simulink library "SDTlibV1"  (R2025b)
settings: Solver=VariableStepAuto  StartTime=0.0  StopTime=10.0  RelTol=1e-3
PreLoadFcn:
  | addpath(genpath('SDTfct'));
values from neighbouring files (symbols this model uses):
  pass = ra2DCMi(blk.ra)    [view_SDTlib_model.m]
undefined symbols (not defined in the file or in its folder): CMG, DAP0, DPa0, FSM, Ignew, InvDyn, InvDynAug, Jr, KIN, kinematic_model, LS, Mdyn, mnew, mp, OGnew, PMA, ra_norm, RWS, sig4, uls, ureal, uss, uw, XI
libraries: RCTblocks x470, $bdroot x4
(part 4 of 10)

== system SDTlibV1/Space  subsystems/Four CMGs Pyramid ==
  Sigma_dot_ref : Inport
  m_at_P : Inport  Port=2
  CMG1 : Subsystem
  CMG2 : Subsystem
  CMG3 : Subsystem
  CMG4 : Subsystem
  Demux : Demux
  Mux : Mux
  P1/p : $bdroot/3//6 dof DCM/6x6 DCM  rot=[cos(CMG.alpha) -sin(CMG.alpha) 0;sin(CMG.alpha) cos(CMG.alpha) 0;0 0 1]*CMG.Pbeta  transp=off
  P1/p' : Subsystem  mask(18x18 Direction cosine matrix (DCM)){rot=[cos(CMG.alpha) -sin(CMG.alpha) 0;sin(CMG.alpha) cos(CMG.alpha) 0;0 0 1]*CMG.Pbeta, transp=on}
      mask prompts: rot "3x3 DCM"; transp "Matrix transposed"
      mask help:
      | For 6 d.o.f. body motion vector (3 translations and 3 rotations, acceleration velocities and positions), this block Implement the 18x18 rotation matrix (or its transposed) for a given 3x3 DCM.
      |
      | Considering 2 frames R1 and  R2, the DCM between R1 and R2 is defined as the 3x3 matrix where each column is the component vector of each R2 orthogonal unit vector expressed in R1. Thus
      |
      |    [v]_R1 = DCM  * [v]_R2.
      mask init:
      | if transp,
      |     rot=rot';
      | end
      mask Help: web('Doc6dcm.html','-browser','-browser')
      mask Display:
      | disp('18x18 DCM')
      | if transp
      |     port_label('input', 1, '[.]_R1')
      |     port_label('output', 1, '[.]_R2')
      | else
      |     port_label('input', 1, '[.]_R2')
      |     port_label('output', 1, '[.]_R1')
      | end
  P2/p : $bdroot/3//6 dof DCM/6x6 DCM  rot=[cos(CMG.alpha+pi/2) -sin(CMG.alpha+pi/2) 0;sin(CMG.alpha+pi/2) cos(CMG.alpha+pi/2) 0;0 0 1]*CMG.Pbeta  transp=off
  P2/p' : Subsystem  mask(18x18 Direction cosine matrix (DCM)){rot=[cos(CMG.alpha+pi/2) -sin(CMG.alpha+pi/2) 0;sin(CMG.alpha+pi/2) cos(CMG.alpha+pi/2) 0;0 0 1]*CMG.Pbeta, transp=on}
      mask prompts: rot "3x3 DCM"; transp "Matrix transposed"
      mask help:
      | For 6 d.o.f. body motion vector (3 translations and 3 rotations, acceleration velocities and positions), this block Implement the 18x18 rotation matrix (or its transposed) for a given 3x3 DCM.
      |
      | Considering 2 frames R1 and  R2, the DCM between R1 and R2 is defined as the 3x3 matrix where each column is the component vector of each R2 orthogonal unit vector expressed in R1. Thus
      |
      |    [v]_R1 = DCM  * [v]_R2.
      mask init:
      | if transp,
      |     rot=rot';
      | end
      mask Help: web('Doc6dcm.html','-browser','-browser')
      mask Display:
      | disp('18x18 DCM')
      | if transp
      |     port_label('input', 1, '[.]_R1')
      |     port_label('output', 1, '[.]_R2')
      | else
      |     port_label('input', 1, '[.]_R2')
      |     port_label('output', 1, '[.]_R1')
      | end
  P3/p : $bdroot/3//6 dof DCM/6x6 DCM  rot=[cos(CMG.alpha+pi) -sin(CMG.alpha+pi) 0;sin(CMG.alpha+pi) cos(CMG.alpha+pi) 0;0 0 1]*CMG.Pbeta  transp=off
  P3/p' : Subsystem  mask(18x18 Direction cosine matrix (DCM)){rot=[cos(CMG.alpha+pi) -sin(CMG.alpha+pi) 0;sin(CMG.alpha+pi) cos(CMG.alpha+pi) 0;0 0 1]*CMG.Pbeta, transp=on}
      mask prompts: rot "3x3 DCM"; transp "Matrix transposed"
      mask help:
      | For 6 d.o.f. body motion vector (3 translations and 3 rotations, acceleration velocities and positions), this block Implement the 18x18 rotation matrix (or its transposed) for a given 3x3 DCM.
      |
      | Considering 2 frames R1 and  R2, the DCM between R1 and R2 is defined as the 3x3 matrix where each column is the component vector of each R2 orthogonal unit vector expressed in R1. Thus
      |
      |    [v]_R1 = DCM  * [v]_R2.
      mask init:
      | if transp,
      |     rot=rot';
      | end
      mask Help: web('Doc6dcm.html','-browser','-browser')
      mask Display:
      | disp('18x18 DCM')
      | if transp
      |     port_label('input', 1, '[.]_R1')
      |     port_label('output', 1, '[.]_R2')
      | else
      |     port_label('input', 1, '[.]_R2')
      |     port_label('output', 1, '[.]_R1')
      | end
  P4/p : $bdroot/3//6 dof DCM/6x6 DCM  rot=[cos(CMG.alpha+3*pi/2) -sin(CMG.alpha+3*pi/2) 0;sin(CMG.alpha+3*pi/2) cos(CMG.alpha+3*pi/2) 0;0 0 1]*CMG.Pbeta  transp=off
  P4/p' : Subsystem  mask(18x18 Direction cosine matrix (DCM)){rot=[cos(CMG.alpha+3*pi/2) -sin(CMG.alpha+3*pi/2) 0;sin(CMG.alpha+3*pi/2) cos(CMG.alpha+3*pi/2) 0;0 0 1]*CMG.Pbeta, transp=on}
      mask prompts: rot "3x3 DCM"; transp "Matrix transposed"
      mask help:
      | For 6 d.o.f. body motion vector (3 translations and 3 rotations, acceleration velocities and positions), this block Implement the 18x18 rotation matrix (or its transposed) for a given 3x3 DCM.
      |
      | Considering 2 frames R1 and  R2, the DCM between R1 and R2 is defined as the 3x3 matrix where each column is the component vector of each R2 orthogonal unit vector expressed in R1. Thus
      |
      |    [v]_R1 = DCM  * [v]_R2.
      mask init:
      | if transp,
      |     rot=rot';
      | end
      mask Help: web('Doc6dcm.html','-browser','-browser')
      mask Display:
      | disp('18x18 DCM')
      | if transp
      |     port_label('input', 1, '[.]_R1')
      |     port_label('output', 1, '[.]_R2')
      | else
      |     port_label('input', 1, '[.]_R2')
      |     port_label('output', 1, '[.]_R1')
      | end
  massless connection body : Subsystem  mask(Massless multi_port [6+18(n-1)]x[6(n-1)+18]){n=5, numinv=5, OP1=[0;-CMG.r;0], OP2=[CMG.r;0;0], OP3=[0;CMG.r;0], OP4=[-CMG.r;0;0], OP5=[0;0;0], OP6=[0;0;0], OP7=[0;0;0]}
      mask prompts: n "Number of ports"; numinv "Port (point) Pj: j="; OP1 "OP1 (3x1 vector, m)"; OP2 "OP2 (3x1 vector, m)"; OP3 "OP3 (3x1 vector, m)"; OP4 "OP4 (3x1 vector, m)"; OP5 "OP5 (3x1 vector,m)"; OP6 "OP6 (3x1 vector,m)"; OP7 "OP7 (3x1 vector,m)"
      mask help:
      | Massless body to transport wrenches and acceleration twists:
      | [6+18(n-1)]x[6(n-1)+18] gain from:
      |  * the motion vector at one point Pj; i.e. the parent port,
      |  * the wrenches applied to this massless body at the n-1 points Pi (i=1,..n, except j); i.e. the child ports
      | to:
      |  * the wrench applied at point Pj by this massless body,
      |  * the motion vectors at the other n-1  points Pi (i=1,..n, except j).
      |
      | 0: the reference point
      | Pi (i=1:n): the n given connection points or ports (1<n<8).
      |
      | All parameters are expressed in the body frame.
      | Each parameter can be an uncertain parameter declared with "ureal"
      mask init:
      | MasslessConnectionBodyAug
      mask Help: %web('DocMassLessBody.html')
      mask TypeOptions n: 2 | 3 | 4 | 5 | 6 | 7
      mask TypeOptions numinv: 1 | 2 | 3 | 4 | 5 | 6 | 7
      mask DialogControl ParameterGroupVar Prompt: Main parameters
      mask DialogControl port1 Prompt: Port #1
      mask DialogControl port2 Prompt: #2
      mask DialogControl port3 Prompt: #3
      mask DialogControl port4 Prompt: #4
      mask DialogControl port5 Prompt: #5
      mask DialogControl port6 Prompt: #6
      mask DialogControl port7 Prompt: #7
      mask Display:
      | disp('Massless\n connection body\n [6+18(n-1)]x[6(n-1)+18]')
      | for ii=1:n+1
      |     if numinv==ii,
      |         port_label('output',ii,['W_body/.,P',num2str(ii)])
      |         port_label('input', ii,['m_P',num2str(ii)])
      |     else
      |         port_label('input', ii,['W_./body,P',num2str(ii)])
      |         port_label('output',ii,['m_P',num2str(ii)])
      |     end
      | end
  Sigma_dot : Outport
  W_CMGs/.,P : Outport  Port=2
  wires:
  Mux/1 -> Sigma_dot/1
  massless connection body/2(out2) -> P2/p'/1(u)
  CMG3/1(W_body/.,P1|p) -> P3/p/1
  P4/p'/1(y) -> CMG4/1(m_P1|p)
  P2/p'/1(y) -> CMG2/1(m_P1|p)
  CMG2/2(sigma_dot) -> Mux/2
  CMG2/1(W_body/.,P1|p) -> P2/p/1
  CMG1/1(W_body/.,P1|p) -> P1/p/1
  P1/p/1 -> massless connection body/1(in1)
  Demux/3 -> CMG3/2(sigma_dot_ref)
  Sigma_dot_ref/1 -> Demux/1
  CMG4/1(W_body/.,P1|p) -> P4/p/1
  CMG4/2(sigma_dot) -> Mux/4
  m_at_P/1 -> massless connection body/5(in5)
  P1/p'/1(y) -> CMG1/1(m_P1|p)
  Demux/2 -> CMG2/2(sigma_dot_ref)
  Demux/4 -> CMG4/2(sigma_dot_ref)
  P4/p/1 -> massless connection body/4(in4)
  P2/p/1 -> massless connection body/2(in2)
  CMG3/2(sigma_dot) -> Mux/3
  massless connection body/4(out4) -> P4/p'/1(u)
  massless connection body/3(out3) -> P3/p'/1(u)
  massless connection body/1(out1) -> P1/p'/1(u)
  Demux/1 -> CMG1/2(sigma_dot_ref)
  P3/p/1 -> massless connection body/3(in3)
  P3/p'/1(y) -> CMG3/1(m_P1|p)
  massless connection body/5(out5) -> W_CMGs/.,P/1
  CMG1/2(sigma_dot) -> Mux/1

== system SDTlibV1/Space  subsystems/RWS ==
  m : Inport  PortDimensions=18
  RW_torque : Inport  Port=2
  RW_dist : Inport  Port=3
  Demux : Demux
  Demux1 : Demux  Outputs=[5 5 5 5]
  Mux : Mux
  RW1 : Subsystem  mask(Actuated/Disturbed reaction wheel (7x24)){ra=RWS.SpinAxis(:,1), m=RWS.m, Iw=RWS.Iw, Ir=RWS.Ir, OG=[0;0;0], OP=[0;0;0], Omega=RWS.w1}
      mask prompts: ra "Wheel axis (3x1 vector)"; m "Wheel mass (Kg)"; Iw "Wheel axial Inertia  (at G, Kgm^2)"; Ir "Wheel radial inertia (at G, Kgm^2)"; OG "OG (3x1 vector, m)"; OP "OP (3x1 vector, m)"; Omega "spinning rate (rd/s)"
      mask help:
      | Dynamic model of a reaction wheel (spinning wheel) at point P (connection point with a parent body):
      | 24x7 transfer from:
      |  * the motion vector at P (18 components)
      |  * the 5 components (3 forces, 2 radial torques) of the wheel induced disturbances (N, Nm)
      |  * the control signal u (Nm) : -u  is applied on the wheel along its spinning axis
      | to:
      |  * the wrench applied by this body at P (6 components).
      |  * the wheel angular acceleration.
      |
      | 0: the reference point
      | G: the center of the wheel
      | P: the connection point
      |
      | All parameters are expressed in the (inherit) body frame.
      | WARNING: the disturbance (input #2) is expressed in the wheel frame.
      | Only the spinning rate can be an uncertain parameter declared with "ureal"
      mask init:
      | pass=ra2DCMi(ra);
      | Tau_GP=kinematic_model(OG,OP);
      mask Help: web('DocRWdist.html','-browser','-browser')
      mask DialogControl ParameterGroupVar Prompt: Main parameters
      mask Display:
      | disp('Reaction wheel\n (7x24)')
      | port_label('input', 1, 'm')
      | port_label('input',2,'Dist: (N,Nm)')
      | port_label('input',3,'u (Nm)')
      | port_label('output', 1, 'W_body/.')
      | port_label('output',2,'\Omega dot (rad/s^2)','interpreter','tex')
  RW2 : Subsystem  mask(Actuated/Disturbed reaction wheel (7x24)){ra=RWS.SpinAxis(:,2), m=RWS.m, Iw=RWS.Iw, Ir=RWS.Ir, OG=[0;0;0], OP=[0;0;0], Omega=RWS.w2}
      mask prompts: ra "Wheel axis (3x1 vector)"; m "Wheel mass (Kg)"; Iw "Wheel axial Inertia  (at G, Kgm^2)"; Ir "Wheel radial inertia (at G, Kgm^2)"; OG "OG (3x1 vector, m)"; OP "OP (3x1 vector, m)"; Omega "spinning rate (rd/s)"
      mask help:
      | Dynamic model of a reaction wheel (spinning wheel) at point P (connection point with a parent body):
      | 24x7 transfer from:
      |  * the motion vector at P (18 components)
      |  * the 5 components (3 forces, 2 radial torques) of the wheel induced disturbances (N, Nm)
      |  * the control signal u (Nm) : -u  is applied on the wheel along its spinning axis
      | to:
      |  * the wrench applied by this body at P (6 components).
      |  * the wheel angular acceleration.
      |
      | 0: the reference point
      | G: the center of the wheel
      | P: the connection point
      |
      | All parameters are expressed in the (inherit) body frame.
      | WARNING: the disturbance (input #2) is expressed in the wheel frame.
      | Only the spinning rate can be an uncertain parameter declared with "ureal"
      mask init:
      | pass=ra2DCMi(ra);
      | Tau_GP=kinematic_model(OG,OP);
      mask Help: web('DocRWdist.html','-browser','-browser')
      mask DialogControl ParameterGroupVar Prompt: Main parameters
      mask Display:
      | disp('Reaction wheel\n (7x24)')
      | port_label('input', 1, 'm')
      | port_label('input',2,'Dist: (N,Nm)')
      | port_label('input',3,'u (Nm)')
      | port_label('output', 1, 'W_body/.')
      | port_label('output',2,'\Omega dot (rad/s^2)','interpreter','tex')
  RW3 : Subsystem  mask(Actuated/Disturbed reaction wheel (7x24)){ra=RWS.SpinAxis(:,3), m=RWS.m, Iw=RWS.Iw, Ir=RWS.Ir, OG=[0;0;0], OP=[0;0;0], Omega=RWS.w3}
      mask prompts: ra "Wheel axis (3x1 vector)"; m "Wheel mass (Kg)"; Iw "Wheel axial Inertia  (at G, Kgm^2)"; Ir "Wheel radial inertia (at G, Kgm^2)"; OG "OG (3x1 vector, m)"; OP "OP (3x1 vector, m)"; Omega "spinning rate (rd/s)"
      mask help:
      | Dynamic model of a reaction wheel (spinning wheel) at point P (connection point with a parent body):
      | 24x7 transfer from:
      |  * the motion vector at P (18 components)
      |  * the 5 components (3 forces, 2 radial torques) of the wheel induced disturbances (N, Nm)
      |  * the control signal u (Nm) : -u  is applied on the wheel along its spinning axis
      | to:
      |  * the wrench applied by this body at P (6 components).
      |  * the wheel angular acceleration.
      |
      | 0: the reference point
      | G: the center of the wheel
      | P: the connection point
      |
      | All parameters are expressed in the (inherit) body frame.
      | WARNING: the disturbance (input #2) is expressed in the wheel frame.
      | Only the spinning rate can be an uncertain parameter declared with "ureal"
      mask init:
      | pass=ra2DCMi(ra);
      | Tau_GP=kinematic_model(OG,OP);
      mask Help: web('DocRWdist.html','-browser','-browser')
      mask DialogControl ParameterGroupVar Prompt: Main parameters
      mask Display:
      | disp('Reaction wheel\n (7x24)')
      | port_label('input', 1, 'm')
      | port_label('input',2,'Dist: (N,Nm)')
      | port_label('input',3,'u (Nm)')
      | port_label('output', 1, 'W_body/.')
      | port_label('output',2,'\Omega dot (rad/s^2)','interpreter','tex')
  RW4 : Subsystem  mask(Actuated/Disturbed reaction wheel (7x24)){ra=RWS.SpinAxis(:,4), m=RWS.m, Iw=RWS.Iw, Ir=RWS.Ir, OG=[0;0;0], OP=[0;0;0], Omega=RWS.w4}
      mask prompts: ra "Wheel axis (3x1 vector)"; m "Wheel mass (Kg)"; Iw "Wheel axial Inertia  (at G, Kgm^2)"; Ir "Wheel radial inertia (at G, Kgm^2)"; OG "OG (3x1 vector, m)"; OP "OP (3x1 vector, m)"; Omega "spinning rate (rd/s)"
      mask help:
      | Dynamic model of a reaction wheel (spinning wheel) at point P (connection point with a parent body):
      | 24x7 transfer from:
      |  * the motion vector at P (18 components)
      |  * the 5 components (3 forces, 2 radial torques) of the wheel induced disturbances (N, Nm)
      |  * the control signal u (Nm) : -u  is applied on the wheel along its spinning axis
      | to:
      |  * the wrench applied by this body at P (6 components).
      |  * the wheel angular acceleration.
      |
      | 0: the reference point
      | G: the center of the wheel
      | P: the connection point
      |
      | All parameters are expressed in the (inherit) body frame.
      | WARNING: the disturbance (input #2) is expressed in the wheel frame.
      | Only the spinning rate can be an uncertain parameter declared with "ureal"
      mask init:
      | pass=ra2DCMi(ra);
      | Tau_GP=kinematic_model(OG,OP);
      mask Help: web('DocRWdist.html','-browser','-browser')
      mask DialogControl ParameterGroupVar Prompt: Main parameters
      mask Display:
      | disp('Reaction wheel\n (7x24)')
      | port_label('input', 1, 'm')
      | port_label('input',2,'Dist: (N,Nm)')
      | port_label('input',3,'u (Nm)')
      | port_label('output', 1, 'W_body/.')
      | port_label('output',2,'\Omega dot (rad/s^2)','interpreter','tex')
  massless connection body : Subsystem  mask(Massless multi_port [6+18(n-1)]x[6(n-1)+18]){n=5, numinv=1, OP1=[0;0;0], OP2=RWS.PC1, OP3=RWS.PC2, OP4=RWS.PC3, OP5=RWS.PC4, OP6=[0;0;0], OP7=[0;0;0]}
      mask prompts: n "Number of ports"; numinv "Port (point) Pj: j="; OP1 "OP1 (3x1 vector, m)"; OP2 "OP2 (3x1 vector, m)"; OP3 "OP3 (3x1 vector, m)"; OP4 "OP4 (3x1 vector, m)"; OP5 "OP5 (3x1 vector,m)"; OP6 "OP6 (3x1 vector,m)"; OP7 "OP7 (3x1 vector,m)"
      mask help:
      | Massless body to transport wrenches and acceleration twists:
      | [6+18(n-1)]x[6(n-1)+18] gain from:
      |  * the motion vector at one point Pj; i.e. the parent port,
      |  * the wrenches applied to this massless body at the n-1 points Pi (i=1,..n, except j); i.e. the child ports
      | to:
      |  * the wrench applied at point Pj by this massless body,
      |  * the motion vectors at the other n-1  points Pi (i=1,..n, except j).
      |
      | 0: the reference point
      | Pi (i=1:n): the n given connection points or ports (1<n<8).
      |
      | All parameters are expressed in the body frame.
      | Each parameter can be an uncertain parameter declared with "ureal"
      mask init:
      | MasslessConnectionBodyAug
      mask Help: %web('DocMassLessBody.html')
      mask TypeOptions n: 2 | 3 | 4 | 5 | 6 | 7
      mask TypeOptions numinv: 1 | 2 | 3 | 4 | 5 | 6 | 7
      mask DialogControl ParameterGroupVar Prompt: Main parameters
      mask DialogControl port1 Prompt: Port #1
      mask DialogControl port2 Prompt: #2
      mask DialogControl port3 Prompt: #3
      mask DialogControl port4 Prompt: #4
      mask DialogControl port5 Prompt: #5
      mask DialogControl port6 Prompt: #6
      mask DialogControl port7 Prompt: #7
      mask Display:
      | disp('Massless\n connection body\n [6+18(n-1)]x[6(n-1)+18]')
      | for ii=1:n+1
      |     if numinv==ii,
      |         port_label('output',ii,['W_body/.,P',num2str(ii)])
      |         port_label('input', ii,['m_P',num2str(ii)])
      |     else
      |         port_label('input', ii,['W_./body,P',num2str(ii)])
      |         port_label('output',ii,['m_P',num2str(ii)])
      |     end
      | end
  W_body/.,P1 : Outport
  RW_acc : Outport  Port=2
  wires:
  RW4/2(Omega_dot) -> Mux/4
  RW3/2(Omega_dot) -> Mux/3
  RW1/2(Omega_dot) -> Mux/1
  Demux/4 -> RW4/3(u (Nm))
  m/1 -> massless connection body/1(in1)
  massless connection body/2(out2) -> RW1/1(m)
  Demux/3 -> RW3/3(u (Nm))
  RW_dist/1 -> Demux1/1
  Demux/1 -> RW1/3(u (Nm))
  RW2/2(Omega_dot) -> Mux/2
  RW2/1(W_body/.) -> massless connection body/3(in3)
  RW4/1(W_body/.) -> massless connection body/5(in5)
  massless connection body/1(out1) -> W_body/.,P1/1
  RW_torque/1 -> Demux/1
  RW1/1(W_body/.) -> massless connection body/2(in2)
  RW3/1(W_body/.) -> massless connection body/4(in4)
  Demux/2 -> RW2/3(u (Nm))
  Mux/1 -> RW_acc/1
  massless connection body/3(out3) -> RW2/1(m)
  massless connection body/4(out4) -> RW3/1(m)
  massless connection body/5(out5) -> RW4/1(m)
  Demux1/1 -> RW1/2("Dist (N, Nm)    ")
  Demux1/2 -> RW2/2("Dist (N, Nm)    ")
  Demux1/3 -> RW3/2("Dist (N, Nm)    ")
  Demux1/4 -> RW4/2("Dist (N, Nm)    ")

== system SDTlibV1/Space  subsystems/Set of 6 PMAss ==
  m_P1 : Inport  PortDimensions=18
  u_PMA : Inport  Port=2
  18x18 DCM : Subsystem  mask(18x18 Direction cosine matrix (DCM)){rot=[1 0 0;0 0 1;0 -1 0], transp=on}
      mask prompts: rot "3x3 DCM"; transp "Matrix transposed"
      mask help:
      | For 6 d.o.f. body motion vector (3 translations and 3 rotations, acceleration velocities and positions), this block Implement the 18x18 rotation matrix (or its transposed) for a given 3x3 DCM.
      |
      | Considering 2 frames R1 and  R2, the DCM between R1 and R2 is defined as the 3x3 matrix where each column is the component vector of each R2 orthogonal unit vector expressed in R1. Thus
      |
      |    [v]_R1 = DCM  * [v]_R2.
      mask init:
      | if transp,
      |     rot=rot';
      | end
      mask Help: web('Doc6dcm.html','-browser','-browser')
      mask Display:
      | disp('18x18 DCM')
      | if transp
      |     port_label('input', 1, '[.]_R1')
      |     port_label('output', 1, '[.]_R2')
      | else
      |     port_label('input', 1, '[.]_R2')
      |     port_label('output', 1, '[.]_R1')
      | end
  18x18 DCM1 : Subsystem  mask(18x18 Direction cosine matrix (DCM)){rot=[1 0 0;0 0 1;0 -1 0]*[cosd(120) 0 -sind(120);0 1 0;sind(120) 0 cosd(120)], transp=on}
      mask prompts: rot "3x3 DCM"; transp "Matrix transposed"
      mask help:
      | For 6 d.o.f. body motion vector (3 translations and 3 rotations, acceleration velocities and positions), this block Implement the 18x18 rotation matrix (or its transposed) for a given 3x3 DCM.
      |
      | Considering 2 frames R1 and  R2, the DCM between R1 and R2 is defined as the 3x3 matrix where each column is the component vector of each R2 orthogonal unit vector expressed in R1. Thus
      |
      |    [v]_R1 = DCM  * [v]_R2.
      mask init:
      | if transp,
      |     rot=rot';
      | end
      mask Help: web('Doc6dcm.html','-browser','-browser')
      mask Display:
      | disp('18x18 DCM')
      | if transp
      |     port_label('input', 1, '[.]_R1')
      |     port_label('output', 1, '[.]_R2')
      | else
      |     port_label('input', 1, '[.]_R2')
      |     port_label('output', 1, '[.]_R1')
      | end
  18x18 DCM2 : Subsystem  mask(18x18 Direction cosine matrix (DCM)){rot=[1 0 0;0 0 1;0 -1 0]*[cosd(240) 0 -sind(240);0 1 0;sind(240) 0 cosd(240)], transp=on}
      mask prompts: rot "3x3 DCM"; transp "Matrix transposed"
      mask help:
      | For 6 d.o.f. body motion vector (3 translations and 3 rotations, acceleration velocities and positions), this block Implement the 18x18 rotation matrix (or its transposed) for a given 3x3 DCM.
      |
      | Considering 2 frames R1 and  R2, the DCM between R1 and R2 is defined as the 3x3 matrix where each column is the component vector of each R2 orthogonal unit vector expressed in R1. Thus
      |
      |    [v]_R1 = DCM  * [v]_R2.
      mask init:
      | if transp,
      |     rot=rot';
      | end
      mask Help: web('Doc6dcm.html','-browser','-browser')
      mask Display:
      | disp('18x18 DCM')
      | if transp
      |     port_label('input', 1, '[.]_R1')
      |     port_label('output', 1, '[.]_R2')
      | else
      |     port_label('input', 1, '[.]_R2')
      |     port_label('output', 1, '[.]_R1')
      | end
  6x6 DCM1 : Subsystem  mask(6x6 Direction cosine matrix (DCM)){rot=[1 0 0;0 0 1;0 -1 0]*[cosd(240) 0 -sind(240);0 1 0;sind(240) 0 cosd(240)], transp=off}
      mask prompts: rot "3x3 DCM"; transp "Matrix transposed"
      mask help:
      | For 6 d.o.f. body motion (3 translations and 3 rotations), this block Implement the 6x6 rotation matrix (or its transposed) for a given 3x3 DCM.
      |
      | Considering 2 frames R1 and  R2, the DCM between R1 and R2 is defined as the 3x3 matrix where each column is the component vector of each R2 orthogonal unit vector expressed in R1. Thus
      |
      |    [v]_R1 = DCM  * [v]_R2.
      mask init:
      | if transp,
      |     rot=rot';
      | end
      mask Help: web('Doc6dcm.html','-browser','-browser')
      mask Display:
      | disp('6x6 DCM')
      | if transp
      |     port_label('input', 1, '[.]_R1')
      |     port_label('output', 1, '[.]_R2')
      | else
      |     port_label('input', 1, '[.]_R2')
      |     port_label('output', 1, '[.]_R1')
      | end
  6x6 DCM2 : Subsystem  mask(6x6 Direction cosine matrix (DCM)){rot=[1 0 0;0 0 1;0 -1 0], transp=off}
      mask prompts: rot "3x3 DCM"; transp "Matrix transposed"
      mask help:
      | For 6 d.o.f. body motion (3 translations and 3 rotations), this block Implement the 6x6 rotation matrix (or its transposed) for a given 3x3 DCM.
      |
      | Considering 2 frames R1 and  R2, the DCM between R1 and R2 is defined as the 3x3 matrix where each column is the component vector of each R2 orthogonal unit vector expressed in R1. Thus
      |
      |    [v]_R1 = DCM  * [v]_R2.
      mask init:
      | if transp,
      |     rot=rot';
      | end
      mask Help: web('Doc6dcm.html','-browser','-browser')
      mask Display:
      | disp('6x6 DCM')
      | if transp
      |     port_label('input', 1, '[.]_R1')
      |     port_label('output', 1, '[.]_R2')
      | else
      |     port_label('input', 1, '[.]_R2')
      |     port_label('output', 1, '[.]_R1')
      | end
  6x6 DCM8 : Subsystem  mask(6x6 Direction cosine matrix (DCM)){rot=[1 0 0;0 0 1;0 -1 0]*[cosd(120) 0 -sind(120);0 1 0;sind(120) 0 cosd(120)], transp=off}
      mask prompts: rot "3x3 DCM"; transp "Matrix transposed"
      mask help:
      | For 6 d.o.f. body motion (3 translations and 3 rotations), this block Implement the 6x6 rotation matrix (or its transposed) for a given 3x3 DCM.
      |
      | Considering 2 frames R1 and  R2, the DCM between R1 and R2 is defined as the 3x3 matrix where each column is the component vector of each R2 orthogonal unit vector expressed in R1. Thus
      |
      |    [v]_R1 = DCM  * [v]_R2.
      mask init:
      | if transp,
      |     rot=rot';
      | end
      mask Help: web('Doc6dcm.html','-browser','-browser')
      mask Display:
      | disp('6x6 DCM')
      | if transp
      |     port_label('input', 1, '[.]_R1')
      |     port_label('output', 1, '[.]_R2')
      | else
      |     port_label('input', 1, '[.]_R2')
      |     port_label('output', 1, '[.]_R1')
      | end
  Demux : Demux  Outputs=6
  Mux1 : Mux  Inputs=6
  PMA1 : Subsystem  mask(Proof mass actuator){Mc=PMA.M, IatG=PMA.IatG, OG=[0;0;PMA.l/2], OP=[0;0;0], v=[0;0;1], mp=PMA.m, k=PMA.k, d=PMA.d}
      mask prompts: Mc "PMA total mass (Kg)"; IatG "PMA total inertia at G (Kgm^2)"; OG "OG (3x1 vector, m)"; OP "OP (3x1 vector, m)"; v "v (3x1 vector)"; mp "Proof mass (Kg)"; k "Stiffness (N/m)"; d "Damper (Ns/m)"
      mask help:
      | 7x19 dynamic model of PMA (Proof Mass Actuator) located at point P (connection point with the hub):
      |   * 6x18 transfer between motion vector at P (Xddoy,P) and wrench applied by the PMA at P (W_body/.,P).
      |   * 1 additional input: the control signal or force (N) applied to the proof mass (u_PMA),
      |   * 1 additional output: the relative position of the proof mass ./. the caging (x_PMA).
      | The model is expressed in the (inherit) body frame.
      |
      | O: refrence point
      | G: CoM of the caging,
      | P: connection point with the parent body
      |
      | v: the direction vector of the spring-mass system.
      | Each parameter (except v) can be an uncertain parameter declared with "ureal"
      mask init:
      | PG=OG-OP;
      mask Help: web('docPMA.html','-browser','-browser')
      mask Display:
      | disp('Proof Mass Actuator \n model(7x19)')
      | port_label('input', 1, 'm_P')
      | port_label('output', 1, 'W_body/.,P')
      | port_label('input', 2, 'u_PMA')
      | port_label('output', 2, 'x_PMA')
  PMA2 : Subsystem  mask(Proof mass actuator){Mc=PMA.M, IatG=PMA.IatG, OG=[0;0;PMA.l/2], OP=[0;0;0], v=[0;0;1], mp=PMA.m, k=PMA.k, d=PMA.d}
      mask prompts: Mc "PMA total mass (Kg)"; IatG "PMA total inertia at G (Kgm^2)"; OG "OG (3x1 vector, m)"; OP "OP (3x1 vector, m)"; v "v (3x1 vector)"; mp "Proof mass (Kg)"; k "Stiffness (N/m)"; d "Damper (Ns/m)"
      mask help:
      | 7x19 dynamic model of PMA (Proof Mass Actuator) located at point P (connection point with the hub):
      |   * 6x18 transfer between motion vector at P (Xddoy,P) and wrench applied by the PMA at P (W_body/.,P).
      |   * 1 additional input: the control signal or force (N) applied to the proof mass (u_PMA),
      |   * 1 additional output: the relative position of the proof mass ./. the caging (x_PMA).
      | The model is expressed in the (inherit) body frame.
      |
      | O: refrence point
      | G: CoM of the caging,
      | P: connection point with the parent body
      |
      | v: the direction vector of the spring-mass system.
      | Each parameter (except v) can be an uncertain parameter declared with "ureal"
      mask init:
      | PG=OG-OP;
      mask Help: web('docPMA.html','-browser','-browser')
      mask Display:
      | disp('Proof Mass Actuator \n model(7x19)')
      | port_label('input', 1, 'm_P')
      | port_label('output', 1, 'W_body/.,P')
      | port_label('input', 2, 'u_PMA')
      | port_label('output', 2, 'x_PMA')
  PMA3 : Subsystem  mask(Proof mass actuator){Mc=PMA.M, IatG=PMA.IatG, OG=[0;0;PMA.l/2], OP=[0;0;0], v=[0;0;1], mp=PMA.m, k=PMA.k, d=PMA.d}
      mask prompts: Mc "PMA total mass (Kg)"; IatG "PMA total inertia at G (Kgm^2)"; OG "OG (3x1 vector, m)"; OP "OP (3x1 vector, m)"; v "v (3x1 vector)"; mp "Proof mass (Kg)"; k "Stiffness (N/m)"; d "Damper (Ns/m)"
      mask help:
      | 7x19 dynamic model of PMA (Proof Mass Actuator) located at point P (connection point with the hub):
      |   * 6x18 transfer between motion vector at P (Xddoy,P) and wrench applied by the PMA at P (W_body/.,P).
      |   * 1 additional input: the control signal or force (N) applied to the proof mass (u_PMA),
      |   * 1 additional output: the relative position of the proof mass ./. the caging (x_PMA).
      | The model is expressed in the (inherit) body frame.
      |
      | O: refrence point
      | G: CoM of the caging,
      | P: connection point with the parent body
      |
      | v: the direction vector of the spring-mass system.
      | Each parameter (except v) can be an uncertain parameter declared with "ureal"
      mask init:
      | PG=OG-OP;
      mask Help: web('docPMA.html','-browser','-browser')
      mask Display:
      | disp('Proof Mass Actuator \n model(7x19)')
      | port_label('input', 1, 'm_P')
      | port_label('output', 1, 'W_body/.,P')
      | port_label('input', 2, 'u_PMA')
      | port_label('output', 2, 'x_PMA')
  PMA4 : Subsystem  mask(Proof mass actuator){Mc=PMA.M, IatG=PMA.IatG, OG=[0;0;PMA.l/2], OP=[0;0;0], v=[0;0;1], mp=PMA.m, k=PMA.k, d=PMA.d}
      mask prompts: Mc "PMA total mass (Kg)"; IatG "PMA total inertia at G (Kgm^2)"; OG "OG (3x1 vector, m)"; OP "OP (3x1 vector, m)"; v "v (3x1 vector)"; mp "Proof mass (Kg)"; k "Stiffness (N/m)"; d "Damper (Ns/m)"
      mask help:
      | 7x19 dynamic model of PMA (Proof Mass Actuator) located at point P (connection point with the hub):
      |   * 6x18 transfer between motion vector at P (Xddoy,P) and wrench applied by the PMA at P (W_body/.,P).
      |   * 1 additional input: the control signal or force (N) applied to the proof mass (u_PMA),
      |   * 1 additional output: the relative position of the proof mass ./. the caging (x_PMA).
      | The model is expressed in the (inherit) body frame.
      |
      | O: refrence point
      | G: CoM of the caging,
      | P: connection point with the parent body
      |
      | v: the direction vector of the spring-mass system.
      | Each parameter (except v) can be an uncertain parameter declared with "ureal"
      mask init:
      | PG=OG-OP;
      mask Help: web('docPMA.html','-browser','-browser')
      mask Display:
      | disp('Proof Mass Actuator \n model(7x19)')
      | port_label('input', 1, 'm_P')
      | port_label('output', 1, 'W_body/.,P')
      | port_label('input', 2, 'u_PMA')
      | port_label('output', 2, 'x_PMA')
  PMA5 : Subsystem  mask(Proof mass actuator){Mc=PMA.M, IatG=PMA.IatG, OG=[0;0;PMA.l/2], OP=[0;0;0], v=[0;0;1], mp=PMA.m, k=PMA.k, d=PMA.d}
      mask prompts: Mc "PMA total mass (Kg)"; IatG "PMA total inertia at G (Kgm^2)"; OG "OG (3x1 vector, m)"; OP "OP (3x1 vector, m)"; v "v (3x1 vector)"; mp "Proof mass (Kg)"; k "Stiffness (N/m)"; d "Damper (Ns/m)"
      mask help:
      | 7x19 dynamic model of PMA (Proof Mass Actuator) located at point P (connection point with the hub):
      |   * 6x18 transfer between motion vector at P (Xddoy,P) and wrench applied by the PMA at P (W_body/.,P).
      |   * 1 additional input: the control signal or force (N) applied to the proof mass (u_PMA),
      |   * 1 additional output: the relative position of the proof mass ./. the caging (x_PMA).
      | The model is expressed in the (inherit) body frame.
      |
      | O: refrence point
      | G: CoM of the caging,
      | P: connection point with the parent body
      |
      | v: the direction vector of the spring-mass system.
      | Each parameter (except v) can be an uncertain parameter declared with "ureal"
      mask init:
      | PG=OG-OP;
      mask Help: web('docPMA.html','-browser','-browser')
      mask Display:
      | disp('Proof Mass Actuator \n model(7x19)')
      | port_label('input', 1, 'm_P')
      | port_label('output', 1, 'W_body/.,P')
      | port_label('input', 2, 'u_PMA')
      | port_label('output', 2, 'x_PMA')
  PMA6 : Subsystem  mask(Proof mass actuator){Mc=PMA.M, IatG=PMA.IatG, OG=[0;0;PMA.l/2], OP=[0;0;0], v=[0;0;1], mp=PMA.m, k=PMA.k, d=PMA.d}
      mask prompts: Mc "PMA total mass (Kg)"; IatG "PMA total inertia at G (Kgm^2)"; OG "OG (3x1 vector, m)"; OP "OP (3x1 vector, m)"; v "v (3x1 vector)"; mp "Proof mass (Kg)"; k "Stiffness (N/m)"; d "Damper (Ns/m)"
      mask help:
      | 7x19 dynamic model of PMA (Proof Mass Actuator) located at point P (connection point with the hub):
      |   * 6x18 transfer between motion vector at P (Xddoy,P) and wrench applied by the PMA at P (W_body/.,P).
      |   * 1 additional input: the control signal or force (N) applied to the proof mass (u_PMA),
      |   * 1 additional output: the relative position of the proof mass ./. the caging (x_PMA).
      | The model is expressed in the (inherit) body frame.
      |
      | O: refrence point
      | G: CoM of the caging,
      | P: connection point with the parent body
      |
      | v: the direction vector of the spring-mass system.
      | Each parameter (except v) can be an uncertain parameter declared with "ureal"
      mask init:
      | PG=OG-OP;
      mask Help: web('docPMA.html','-browser','-browser')
      mask Display:
      | disp('Proof Mass Actuator \n model(7x19)')
      | port_label('input', 1, 'm_P')
      | port_label('output', 1, 'W_body/.,P')
      | port_label('input', 2, 'u_PMA')
      | port_label('output', 2, 'x_PMA')
  massless connection body : Subsystem  mask(Massless multi_port [6+18(n-1)]x[6(n-1)+18]){n=7, numinv=1, OP1=[0;0;0], OP2=PMA.r*[cosd(0)     sind(0)     0]', OP3=PMA.r*[cosd(120)   sind(120)   0]', OP4=PMA.r*[cosd(240)   sind(240)   0]', OP5=PMA.r*[cosd(0)     sind(0)     0]', OP6=PMA.r*[cosd(120)   sind(120)   0]', OP7=PMA.r*[cosd(240)   sind(240)   0]'}
      mask prompts: n "Number of ports"; numinv "Port (point) Pj: j="; OP1 "OP1 (3x1 vector, m)"; OP2 "OP2 (3x1 vector, m)"; OP3 "OP3 (3x1 vector, m)"; OP4 "OP4 (3x1 vector, m)"; OP5 "OP5 (3x1 vector,m)"; OP6 "OP6 (3x1 vector,m)"; OP7 "OP7 (3x1 vector,m)"
      mask help:
      | Massless body to transport wrenches and acceleration twists:
      | [6+18(n-1)]x[6(n-1)+18] gain from:
      |  * the motion vector at one point Pj; i.e. the parent port,
      |  * the wrenches applied to this massless body at the n-1 points Pi (i=1,..n, except j); i.e. the child ports
      | to:
      |  * the wrench applied at point Pj by this massless body,
      |  * the motion vectors at the other n-1  points Pi (i=1,..n, except j).
      |
      | 0: the reference point
      | Pi (i=1:n): the n given connection points or ports (1<n<8).
      |
      | All parameters are expressed in the body frame.
      | Each parameter can be an uncertain parameter declared with "ureal"
      mask init:
      | MasslessConnectionBodyAug
      mask Help: %web('DocMassLessBody.html')
      mask TypeOptions n: 2 | 3 | 4 | 5 | 6 | 7
      mask TypeOptions numinv: 1 | 2 | 3 | 4 | 5 | 6 | 7
      mask DialogControl ParameterGroupVar Prompt: Main parameters
      mask DialogControl port1 Prompt: Port #1
      mask DialogControl port2 Prompt: #2
      mask DialogControl port3 Prompt: #3
      mask DialogControl port4 Prompt: #4
      mask DialogControl port5 Prompt: #5
      mask DialogControl port6 Prompt: #6
      mask DialogControl port7 Prompt: #7
      mask Display:
      | disp('Massless\n connection body\n [6+18(n-1)]x[6(n-1)+18]')
      | for ii=1:n+1
      |     if numinv==ii,
      |         port_label('output',ii,['W_body/.,P',num2str(ii)])
      |         port_label('input', ii,['m_P',num2str(ii)])
      |     else
      |         port_label('input', ii,['W_./body,P',num2str(ii)])
      |         port_label('output',ii,['m_P',num2str(ii)])
      |     end
      | end
  W_body/.,P1 : Outport
  x_PMA : Outport  Port=2
  wires:
  massless connection body/2(out2) -> PMA1/1(m_P)
  massless connection body/4(out4) -> PMA3/1(m_P)
  PMA5/1(W_body/.,P) -> 6x6 DCM8/1(u)
  Demux/5 -> PMA5/2(u_PMA)
  Demux/1 -> PMA1/2(u_PMA)
  PMA4/2(x_PMA) -> Mux1/4
  Demux/4 -> PMA4/2(u_PMA)
  massless connection body/6(out6) -> 18x18 DCM1/1(u)
  m_P1/1 -> massless connection body/1(in1)
  PMA5/2(x_PMA) -> Mux1/5
  PMA3/2(x_PMA) -> Mux1/3
  u_PMA/1 -> Demux/1
  PMA6/2(x_PMA) -> Mux1/6
  PMA2/2(x_PMA) -> Mux1/2
  Demux/6 -> PMA6/2(u_PMA)
  Mux1/1 -> x_PMA/1
  massless connection body/1(out1) -> W_body/.,P1/1
  PMA4/1(W_body/.,P) -> 6x6 DCM2/1(u)
  massless connection body/5(out5) -> 18x18 DCM/1(u)
  PMA3/1(W_body/.,P) -> massless connection body/4(in4)
  PMA1/2(x_PMA) -> Mux1/1
  Demux/3 -> PMA3/2(u_PMA)
  PMA2/1(W_body/.,P) -> massless connection body/3(in3)
  Demux/2 -> PMA2/2(u_PMA)
  massless connection body/7(out7) -> 18x18 DCM2/1(u)
  massless connection body/3(out3) -> PMA2/1(m_P)
  PMA1/1(W_body/.,P) -> massless connection body/2(in2)
  PMA6/1(W_body/.,P) -> 6x6 DCM1/1(u)
  6x6 DCM8/1(y) -> massless connection body/6(in6)
  6x6 DCM1/1(y) -> massless connection body/7(in7)
  6x6 DCM2/1(y) -> massless connection body/5(in5)
  18x18 DCM2/1(y) -> PMA6/1(m_P)
  18x18 DCM1/1(y) -> PMA5/1(m_P)
  18x18 DCM/1(y) -> PMA4/1(m_P)

== system SDTlibV1/3//6//18 DCM/18x18 v-u_rotation/Subsystem ==
  In1 : Inport
  Demux : Demux  Outputs=3
  Gain : Gain  Gain=2
  Gain1 : Gain  Gain=-2
  Gain2 : Gain  Gain=2
  Gain3 : Gain  Gain=2
  Gain4 : Gain  Gain=pass  Multiplication=Matrix(K*u) (u vector)
  Gain5 : Gain  Gain=pass'  Multiplication=Matrix(K*u) (u vector)
  Mux : Mux  Inputs=3
  Sum : Sum  Inputs=++|
  Sum1 : Sum  Inputs=|++
  Sum2 : Sum  Inputs=|+-
  Sum3 : Sum  Inputs=|++
  Sum4 : Sum  Inputs=++|
  Sum5 : Sum  Inputs=++|
  Uncertain State Space{,1..3} (4 alike) : RCTblocks/Uncertain State Space  Tag=USS  USystem=uss(sig4)  UValue=[]  X0=[]  uX0=[]
  Out1 : Outport  VectorParamsAs1DForOutWhenUnconnected=off
  wires:
  Gain5/1 -> Demux/1
  Gain4/1 -> Out1/1
  Uncertain State Space3/1 -> Sum3/2
  Gain2/1 -> Sum3/1
  In1/1 -> Gain5/1
  Gain/1 -> Sum/2
  Uncertain State Space2/1 -> Uncertain State Space3/1, Sum4/2, Sum2/2
  Demux/1 -> Gain3/1, Sum1/2
  Demux/3 -> Mux/3
  Mux/1 -> Gain4/1
  Sum4/1 -> Mux/2
  Sum3/1 -> Uncertain State Space2/1
  Gain1/1 -> Sum2/1
  Uncertain State Space/1 -> Uncertain State Space1/1, Sum5/1, Sum1/1
  Gain3/1 -> Sum5/2
  Sum/1 -> Uncertain State Space/1
  Demux/2 -> Sum4/1, Gain1/1
  Uncertain State Space1/1 -> Sum/1
  Sum2/1 -> Gain/1
  Sum1/1 -> Mux/1
  Sum5/1 -> Gain2/1

== system SDTlibV1/3//6//18 DCM/18x18 v-u_rotation/Subsystem1 ==
  In1 : Inport
  Demux : Demux  Outputs=3
  Gain : Gain  Gain=2
  Gain1 : Gain  Gain=-2
  Gain2 : Gain  Gain=2
  Gain3 : Gain  Gain=2
  Gain4 : Gain  Gain=pass  Multiplication=Matrix(K*u) (u vector)
  Gain5 : Gain  Gain=pass'  Multiplication=Matrix(K*u) (u vector)
  Mux : Mux  Inputs=3
  Sum : Sum  Inputs=++|
  Sum1 : Sum  Inputs=|++
  Sum2 : Sum  Inputs=|+-
  Sum3 : Sum  Inputs=|++
  Sum4 : Sum  Inputs=++|
  Sum5 : Sum  Inputs=++|
  Uncertain State Space{,1..3} (4 alike) : RCTblocks/Uncertain State Space  Tag=USS  USystem=uss(sig4)  UValue=[]  X0=[]  uX0=[]
  Out1 : Outport  VectorParamsAs1DForOutWhenUnconnected=off
  wires:
  Gain5/1 -> Demux/1
  Sum5/1 -> Gain2/1
  Sum1/1 -> Mux/1
  Sum2/1 -> Gain/1
  Uncertain State Space1/1 -> Sum/1
  Demux/2 -> Gain1/1, Sum4/1
  Sum/1 -> Uncertain State Space/1
  Gain3/1 -> Sum5/2
  Uncertain State Space/1 -> Sum1/1, Sum5/1, Uncertain State Space1/1
  Gain1/1 -> Sum2/1
  Sum3/1 -> Uncertain State Space2/1
  Sum4/1 -> Mux/2
  Mux/1 -> Gain4/1
  Demux/3 -> Mux/3
  Demux/1 -> Sum1/2, Gain3/1
  Uncertain State Space2/1 -> Sum2/2, Sum4/2, Uncertain State Space3/1
  Gain/1 -> Sum/2
  In1/1 -> Gain5/1
  Gain2/1 -> Sum3/1
  Uncertain State Space3/1 -> Sum3/2
  Gain4/1 -> Out1/1

== system SDTlibV1/3//6//18 DCM/18x18 v-u_rotation/Subsystem2 ==
  In1 : Inport
  Demux : Demux  Outputs=3
  Gain : Gain  Gain=2
  Gain1 : Gain  Gain=-2
  Gain2 : Gain  Gain=2
  Gain3 : Gain  Gain=2
  Gain4 : Gain  Gain=pass  Multiplication=Matrix(K*u) (u vector)
  Gain5 : Gain  Gain=pass'  Multiplication=Matrix(K*u) (u vector)
  Mux : Mux  Inputs=3
  Sum : Sum  Inputs=++|
  Sum1 : Sum  Inputs=|++
  Sum2 : Sum  Inputs=|+-
  Sum3 : Sum  Inputs=|++
  Sum4 : Sum  Inputs=++|
  Sum5 : Sum  Inputs=++|
  Uncertain State Space{,1..3} (4 alike) : RCTblocks/Uncertain State Space  Tag=USS  USystem=uss(sig4)  UValue=[]  X0=[]  uX0=[]
  Out1 : Outport  VectorParamsAs1DForOutWhenUnconnected=off
  wires:
  Sum5/1 -> Gain2/1
  Sum1/1 -> Mux/1
  Sum2/1 -> Gain/1
  Uncertain State Space1/1 -> Sum/1
  Demux/2 -> Gain1/1, Sum4/1
  Sum/1 -> Uncertain State Space/1
  Gain3/1 -> Sum5/2
  Uncertain State Space/1 -> Sum1/1, Sum5/1, Uncertain State Space1/1
  Gain1/1 -> Sum2/1
  Sum3/1 -> Uncertain State Space2/1
  Sum4/1 -> Mux/2
  Mux/1 -> Gain4/1
  Demux/3 -> Mux/3
  Demux/1 -> Sum1/2, Gain3/1
  Uncertain State Space2/1 -> Sum2/2, Sum4/2, Uncertain State Space3/1
  Gain/1 -> Sum/2
  In1/1 -> Gain5/1
  Gain2/1 -> Sum3/1
  Uncertain State Space3/1 -> Sum3/2
  Gain4/1 -> Out1/1
  Gain5/1 -> Demux/1

== system SDTlibV1/3//6//18 DCM/18x18 v-u_rotation/Subsystem3 ==
  In1 : Inport
  Demux : Demux  Outputs=3
  Gain : Gain  Gain=2
  Gain1 : Gain  Gain=-2
  Gain2 : Gain  Gain=2
  Gain3 : Gain  Gain=2
  Gain4 : Gain  Gain=pass  Multiplication=Matrix(K*u) (u vector)
  Gain5 : Gain  Gain=pass'  Multiplication=Matrix(K*u) (u vector)
  Mux : Mux  Inputs=3
  Sum : Sum  Inputs=++|
  Sum1 : Sum  Inputs=|++
  Sum2 : Sum  Inputs=|+-
  Sum3 : Sum  Inputs=|++
  Sum4 : Sum  Inputs=++|
  Sum5 : Sum  Inputs=++|
  Uncertain State Space{,1..3} (4 alike) : RCTblocks/Uncertain State Space  Tag=USS  USystem=uss(sig4)  UValue=[]  X0=[]  uX0=[]
  Out1 : Outport  VectorParamsAs1DForOutWhenUnconnected=off
  wires:
  Gain4/1 -> Out1/1
  Uncertain State Space3/1 -> Sum3/2
  Gain2/1 -> Sum3/1
  In1/1 -> Gain5/1
  Gain/1 -> Sum/2
  Uncertain State Space2/1 -> Uncertain State Space3/1, Sum4/2, Sum2/2
  Demux/1 -> Gain3/1, Sum1/2
  Demux/3 -> Mux/3
  Mux/1 -> Gain4/1
  Sum4/1 -> Mux/2
  Sum3/1 -> Uncertain State Space2/1
  Gain1/1 -> Sum2/1
  Uncertain State Space/1 -> Uncertain State Space1/1, Sum5/1, Sum1/1
  Gain3/1 -> Sum5/2
  Sum/1 -> Uncertain State Space/1
  Demux/2 -> Sum4/1, Gain1/1
  Uncertain State Space1/1 -> Sum/1
  Sum2/1 -> Gain/1
  Sum1/1 -> Mux/1
  Sum5/1 -> Gain2/1
  Gain5/1 -> Demux/1

== system SDTlibV1/3//6//18 DCM/18x18 v-u_rotation/Subsystem4 ==
  In1 : Inport
  Demux : Demux  Outputs=3
  Gain : Gain  Gain=2
  Gain1 : Gain  Gain=-2
  Gain2 : Gain  Gain=2
  Gain3 : Gain  Gain=2
  Gain4 : Gain  Gain=pass  Multiplication=Matrix(K*u) (u vector)
  Gain5 : Gain  Gain=pass'  Multiplication=Matrix(K*u) (u vector)
  Mux : Mux  Inputs=3
  Sum : Sum  Inputs=++|
  Sum1 : Sum  Inputs=|++
  Sum2 : Sum  Inputs=|+-
  Sum3 : Sum  Inputs=|++
  Sum4 : Sum  Inputs=++|
  Sum5 : Sum  Inputs=++|
  Uncertain State Space{,1..3} (4 alike) : RCTblocks/Uncertain State Space  Tag=USS  USystem=uss(sig4)  UValue=[]  X0=[]  uX0=[]
  Out1 : Outport  VectorParamsAs1DForOutWhenUnconnected=off
  wires:
  Gain5/1 -> Demux/1
  Gain4/1 -> Out1/1
  Uncertain State Space3/1 -> Sum3/2
  Gain2/1 -> Sum3/1
  In1/1 -> Gain5/1
  Gain/1 -> Sum/2
  Uncertain State Space2/1 -> Uncertain State Space3/1, Sum4/2, Sum2/2
  Demux/1 -> Gain3/1, Sum1/2
  Demux/3 -> Mux/3
  Mux/1 -> Gain4/1
  Sum4/1 -> Mux/2
  Sum3/1 -> Uncertain State Space2/1
  Gain1/1 -> Sum2/1
  Uncertain State Space/1 -> Uncertain State Space1/1, Sum5/1, Sum1/1
  Gain3/1 -> Sum5/2
  Sum/1 -> Uncertain State Space/1
  Demux/2 -> Sum4/1, Gain1/1
  Uncertain State Space1/1 -> Sum/1
  Sum2/1 -> Gain/1
  Sum1/1 -> Mux/1
  Sum5/1 -> Gain2/1

== system SDTlibV1/3//6//18 DCM/18x18 v-u_rotation/Subsystem5 ==
  In1 : Inport
  Demux : Demux  Outputs=3
  Gain : Gain  Gain=2
  Gain1 : Gain  Gain=-2
  Gain2 : Gain  Gain=2
  Gain3 : Gain  Gain=2
  Gain4 : Gain  Gain=pass  Multiplication=Matrix(K*u) (u vector)
  Gain5 : Gain  Gain=pass'  Multiplication=Matrix(K*u) (u vector)
  Mux : Mux  Inputs=3
  Sum : Sum  Inputs=++|
  Sum1 : Sum  Inputs=|++
  Sum2 : Sum  Inputs=|+-
  Sum3 : Sum  Inputs=|++
  Sum4 : Sum  Inputs=++|
  Sum5 : Sum  Inputs=++|
  Uncertain State Space{,1..3} (4 alike) : RCTblocks/Uncertain State Space  Tag=USS  USystem=uss(sig4)  UValue=[]  X0=[]  uX0=[]
  Out1 : Outport  VectorParamsAs1DForOutWhenUnconnected=off
  wires:
  Gain5/1 -> Demux/1
  Sum5/1 -> Gain2/1
  Sum1/1 -> Mux/1
  Sum2/1 -> Gain/1
  Uncertain State Space1/1 -> Sum/1
  Demux/2 -> Gain1/1, Sum4/1
  Sum/1 -> Uncertain State Space/1
  Gain3/1 -> Sum5/2
  Uncertain State Space/1 -> Sum1/1, Sum5/1, Uncertain State Space1/1
  Gain1/1 -> Sum2/1
  Sum3/1 -> Uncertain State Space2/1
  Sum4/1 -> Mux/2
  Mux/1 -> Gain4/1
  Demux/3 -> Mux/3
  Demux/1 -> Sum1/2, Gain3/1
  Uncertain State Space2/1 -> Sum2/2, Sum4/2, Uncertain State Space3/1
  Gain/1 -> Sum/2
  In1/1 -> Gain5/1
  Gain2/1 -> Sum3/1
  Uncertain State Space3/1 -> Sum3/2
  Gain4/1 -> Out1/1

== system SDTlibV1/3//6//18 DCM/6x6 v-u_rotation/Subsystem ==
  In1 : Inport
  Demux : Demux  Outputs=3
  Gain : Gain  Gain=2
  Gain1 : Gain  Gain=-2
  Gain2 : Gain  Gain=2
  Gain3 : Gain  Gain=2
  Gain4 : Gain  Gain=pass  Multiplication=Matrix(K*u) (u vector)
  Gain5 : Gain  Gain=pass'  Multiplication=Matrix(K*u) (u vector)
  Mux : Mux  Inputs=3
  Sum : Sum  Inputs=++|
  Sum1 : Sum  Inputs=|++
  Sum2 : Sum  Inputs=|+-
  Sum3 : Sum  Inputs=|++
  Sum4 : Sum  Inputs=++|
  Sum5 : Sum  Inputs=++|
  Uncertain State Space{,1..3} (4 alike) : RCTblocks/Uncertain State Space  Tag=USS  USystem=uss(sig4)  UValue=[]  X0=[]  uX0=[]
  Out1 : Outport  VectorParamsAs1DForOutWhenUnconnected=off
  wires:
  Sum5/1 -> Gain2/1
  Sum1/1 -> Mux/1
  Sum2/1 -> Gain/1
  Uncertain State Space1/1 -> Sum/1
  Demux/2 -> Gain1/1, Sum4/1
  Sum/1 -> Uncertain State Space/1
  Gain3/1 -> Sum5/2
  Uncertain State Space/1 -> Sum1/1, Sum5/1, Uncertain State Space1/1
  Gain1/1 -> Sum2/1
  Sum3/1 -> Uncertain State Space2/1
  Sum4/1 -> Mux/2
  Mux/1 -> Gain4/1
  Demux/3 -> Mux/3
  Demux/1 -> Sum1/2, Gain3/1
  Uncertain State Space2/1 -> Sum2/2, Sum4/2, Uncertain State Space3/1
  Gain/1 -> Sum/2
  In1/1 -> Gain5/1
  Gain2/1 -> Sum3/1
  Uncertain State Space3/1 -> Sum3/2
  Gain4/1 -> Out1/1
  Gain5/1 -> Demux/1

== system SDTlibV1/3//6//18 DCM/6x6 v-u_rotation/Subsystem1 ==
  In1 : Inport
  Demux : Demux  Outputs=3
  Gain : Gain  Gain=2
  Gain1 : Gain  Gain=-2
  Gain2 : Gain  Gain=2
  Gain3 : Gain  Gain=2
  Gain4 : Gain  Gain=pass  Multiplication=Matrix(K*u) (u vector)
  Gain5 : Gain  Gain=pass'  Multiplication=Matrix(K*u) (u vector)
  Mux : Mux  Inputs=3
  Sum : Sum  Inputs=++|
  Sum1 : Sum  Inputs=|++
  Sum2 : Sum  Inputs=|+-
  Sum3 : Sum  Inputs=|++
  Sum4 : Sum  Inputs=++|
  Sum5 : Sum  Inputs=++|
  Uncertain State Space{,1..3} (4 alike) : RCTblocks/Uncertain State Space  Tag=USS  USystem=uss(sig4)  UValue=[]  X0=[]  uX0=[]
  Out1 : Outport  VectorParamsAs1DForOutWhenUnconnected=off
  wires:
  Gain4/1 -> Out1/1
  Uncertain State Space3/1 -> Sum3/2
  Gain2/1 -> Sum3/1
  In1/1 -> Gain5/1
  Gain/1 -> Sum/2
  Uncertain State Space2/1 -> Uncertain State Space3/1, Sum4/2, Sum2/2
  Demux/1 -> Gain3/1, Sum1/2
  Demux/3 -> Mux/3
  Mux/1 -> Gain4/1
  Sum4/1 -> Mux/2
  Sum3/1 -> Uncertain State Space2/1
  Gain1/1 -> Sum2/1
  Uncertain State Space/1 -> Uncertain State Space1/1, Sum5/1, Sum1/1
  Gain3/1 -> Sum5/2
  Sum/1 -> Uncertain State Space/1
  Demux/2 -> Sum4/1, Gain1/1
  Uncertain State Space1/1 -> Sum/1
  Sum2/1 -> Gain/1
  Sum1/1 -> Mux/1
  Sum5/1 -> Gain2/1
  Gain5/1 -> Demux/1

== system SDTlibV1/3//6//18 DCM/6x6 z-u_rotation/Subsystem ==
  In1 : Inport
  Demux1 : Demux  Outputs=3
  Gain : Gain  Gain=2
  Gain1 : Gain  Gain=-2
  Gain2 : Gain  Gain=2
  Gain3 : Gain  Gain=2
  Mux1 : Mux  Inputs=3
  Sum : Sum  Inputs=++|
  Sum1 : Sum  Inputs=|++
  Sum2 : Sum  Inputs=|+-
  Sum3 : Sum  Inputs=|++
  Sum4 : Sum  Inputs=++|
  Sum5 : Sum  Inputs=++|
  Uncertain State Space{,1..3} (4 alike) : RCTblocks/Uncertain State Space  Tag=USS  USystem=uss(sig4)  UValue=[]  X0=[]  uX0=[]
  Out1 : Outport  VectorParamsAs1DForOutWhenUnconnected=off
  wires:
  In1/1 -> Demux1/1
  Uncertain State Space3/1 -> Sum3/2
  Sum4/1 -> Mux1/2
  Demux1/2 -> Sum4/1, Gain1/1
  Sum2/1 -> Gain/1
  Sum/1 -> Uncertain State Space/1
  Uncertain State Space2/1 -> Sum2/2, Sum4/2, Uncertain State Space3/1
  Sum3/1 -> Uncertain State Space2/1
  Gain1/1 -> Sum2/1
  Sum5/1 -> Gain2/1
  Demux1/3 -> Mux1/3
  Demux1/1 -> Sum1/2, Gain3/1
  Gain2/1 -> Sum3/1
  Mux1/1 -> Out1/1
  Gain3/1 -> Sum5/2
  Uncertain State Space1/1 -> Sum/1
  Uncertain State Space/1 -> Sum1/1, Sum5/1, Uncertain State Space1/1
  Gain/1 -> Sum/2
  Sum1/1 -> Mux1/1

== system SDTlibV1/3//6//18 DCM/6x6 z-u_rotation/Subsystem1 ==
  In1 : Inport
  Demux1 : Demux  Outputs=3
  Gain : Gain  Gain=2
  Gain1 : Gain  Gain=-2
  Gain2 : Gain  Gain=2
  Gain3 : Gain  Gain=2
  Mux1 : Mux  Inputs=3
  Sum : Sum  Inputs=++|
  Sum1 : Sum  Inputs=|++
  Sum2 : Sum  Inputs=|+-
  Sum3 : Sum  Inputs=|++
  Sum4 : Sum  Inputs=++|
  Sum5 : Sum  Inputs=++|
  Uncertain State Space{,1..3} (4 alike) : RCTblocks/Uncertain State Space  Tag=USS  USystem=uss(sig4)  UValue=[]  X0=[]  uX0=[]
  Out1 : Outport  VectorParamsAs1DForOutWhenUnconnected=off
  wires:
  Sum1/1 -> Mux1/1
  Gain/1 -> Sum/2
  Uncertain State Space/1 -> Uncertain State Space1/1, Sum5/1, Sum1/1
  Uncertain State Space1/1 -> Sum/1
  Gain3/1 -> Sum5/2
  Mux1/1 -> Out1/1
  Gain2/1 -> Sum3/1
  Demux1/1 -> Gain3/1, Sum1/2
  Demux1/3 -> Mux1/3
  Sum5/1 -> Gain2/1
  Gain1/1 -> Sum2/1
  Sum3/1 -> Uncertain State Space2/1
  Uncertain State Space2/1 -> Uncertain State Space3/1, Sum4/2, Sum2/2
  Sum/1 -> Uncertain State Space/1
  Sum2/1 -> Gain/1
  Demux1/2 -> Gain1/1, Sum4/1
  Sum4/1 -> Mux1/2
  Uncertain State Space3/1 -> Sum3/2
  In1/1 -> Demux1/1

== system SDTlibV1/6 dof mechanisms/PMA/Multi port rigid body ==
  in1 : Inport  PortDimensions=18
  in2 : Inport  Port=2  PortDimensions=6
  Demux : Demux  Outputs=[ 6 18]
  Gain : RCTblocks/Uncertain State Space  Tag=USS  USystem=uss(InvDynAug)  UValue=[]  X0=[]  uX0=[]
  Mux : Mux  Inputs=[ 18 6]
  out1 : Outport
  out2 : Outport  Port=2
  wires:
  Mux/1 -> Gain/1
  Gain/1 -> Demux/1
  in1/1 -> Mux/1
  Demux/1 -> out1/1
  in2/1 -> Mux/2
  Demux/2 -> out2/1
